simulink model "p2"  (R2024b)
settings: Solver=VariableStepAuto  StartTime=0.0  StopTime=10.0  RelTol=1e-3
settings Model: Creator=Borjazz  LastModifiedBy=Borjazz

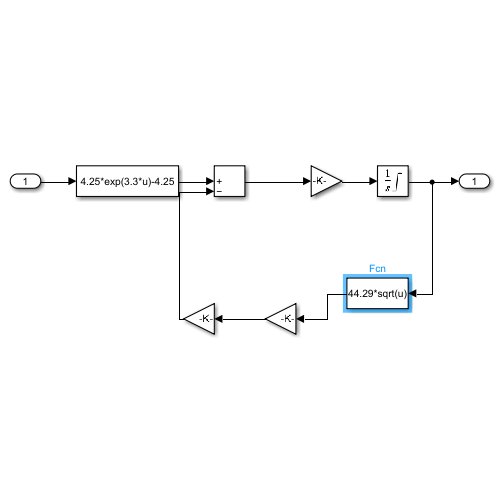
[thumbnail: Simulink's stored preview of the top-level diagram]
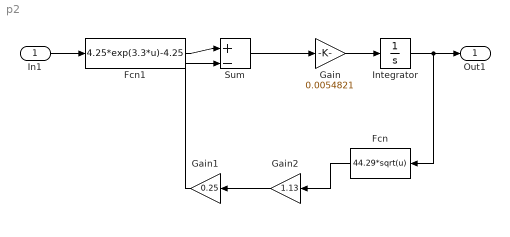
== system p2 ==
  In1 : Inport
  Fcn : Fcn  Expr=44.29*sqrt(u)
  Fcn1 : Fcn  Expr=4.25*exp(3.3*u)-4.25
  Gain : Gain  Gain=0.0054821
  Gain1 : Gain  Gain=0.25
  Gain2 : Gain  Gain=1.13
  Integrator : Integrator  InitialCondition=15  LimitOutput=on  UpperSaturationLimit=78  LowerSaturationLimit=-0
  Sum : Sum  Inputs=|+-
  Out1 : Outport
  wires:
  In1/1 -> Fcn1/1
  Fcn1/1 -> Sum/1
  Sum/1 -> Gain/1
  Gain/1 -> Integrator/1
  Integrator/1 -> Fcn/1, Out1/1
  Fcn/1 -> Gain2/1
  Gain2/1 -> Gain1/1
  Gain1/1 -> Sum/2
